simulink model "Motor_Model"  (R2025b)
settings: Solver=VariableStepAuto  StartTime=0.0  StopTime=2  RelTol=1e-3
undefined symbols (not defined in the file): c, J1, J2, k, ke, km, L, Mc, Ms, R

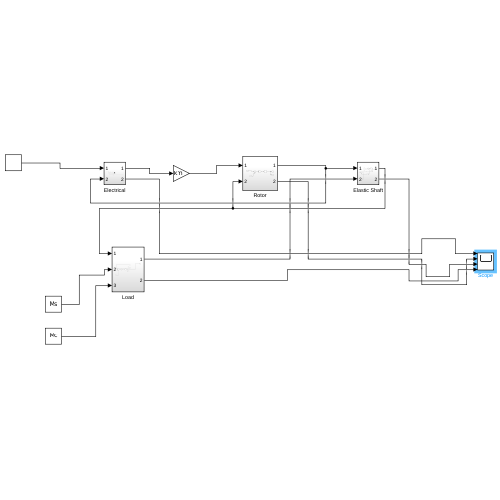
[thumbnail: Simulink's stored preview of the top-level diagram]
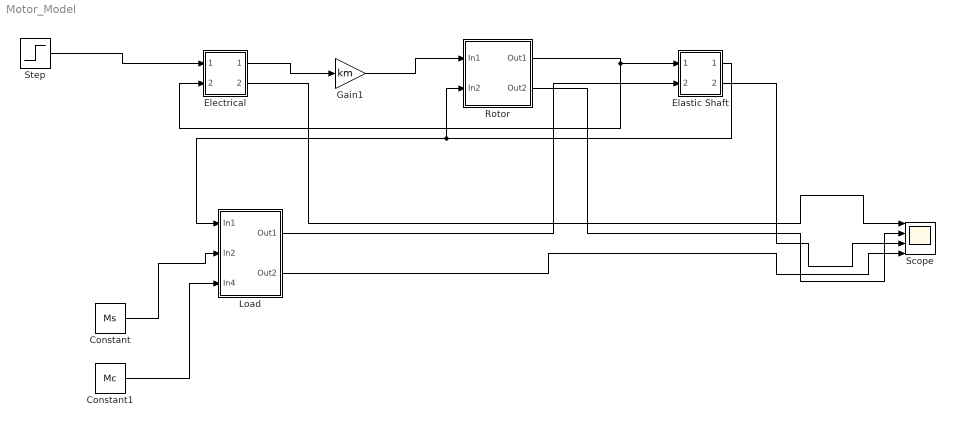
== system Motor_Model ==
  Constant : Constant  Value=Ms
  Constant1 : Constant  Value=Mc
  Elastic Shaft : Subsystem
  Electrical : Subsystem
  Gain1 : Gain  Gain=km
  Load : Subsystem
  Rotor : Subsystem
  Scope : Scope  NumInputPorts=4
      settings: ActiveDisplayYMinimum=-1.1593735821499702  ActiveDisplayYMaximum=10.434362239349735
  Step : Step  Time=0  After=24  SampleTime=0
  wires:
  Step/1 -> Electrical/1(In1)
  Electrical/1(Out1) -> Gain1/1
  Rotor/1(Out1) -> Electrical/2(In2), Elastic Shaft/1(In1)
  Gain1/1 -> Rotor/1(In1)
  Elastic Shaft/1(Out1) -> Load/1(In1), Rotor/2(In2)
  Load/1(Out1) -> Elastic Shaft/2(In2)
  Constant/1 -> Load/2(In2)
  Constant1/1 -> Load/3(In4)
  Electrical/2(Out2) -> Scope/1
  Rotor/2(Out2) -> Scope/2
  Elastic Shaft/2(Out3) -> Scope/3
  Load/2(Out2) -> Scope/4

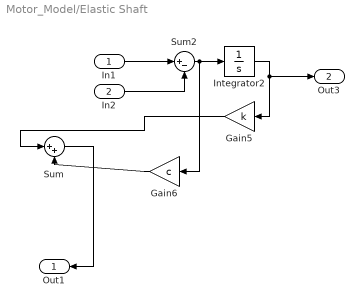
== system Motor_Model/Elastic Shaft ==
  In1 : Inport
  In2 : Inport  Port=2
  Gain5 : Gain  Gain=k
  Gain6 : Gain  Gain=c
  Integrator2 : Integrator
  Sum : Sum  Inputs=|++
  Sum2 : Sum  Inputs=|+-
  Out1 : Outport
  Out3 : Outport  Port=2
  wires:
  Sum2/1 -> Gain6/1, Integrator2/1
  In1/1 -> Sum2/1
  Integrator2/1 -> Out3/1, Gain5/1
  In2/1 -> Sum2/2
  Gain6/1 -> Sum/2
  Sum/1 -> Out1/1
  Gain5/1 -> Sum/1

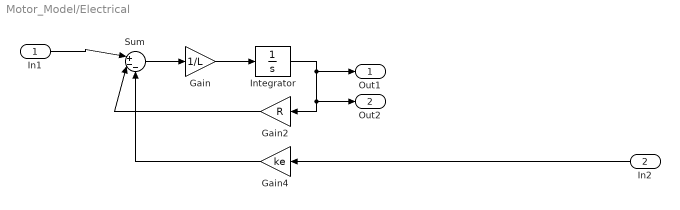
== system Motor_Model/Electrical ==
  In1 : Inport
  In2 : Inport  Port=2
  Gain : Gain  Gain=1/L
  Gain2 : Gain  Gain=R
  Gain4 : Gain  Gain=ke
  Integrator : Integrator
  Sum : Sum  Inputs=|+--
  Out1 : Outport
  Out2 : Outport  Port=2
  wires:
  Gain2/1 -> Sum/2
  Gain4/1 -> Sum/3
  Sum/1 -> Gain/1
  Gain/1 -> Integrator/1
  In2/1 -> Gain4/1
  In1/1 -> Sum/1
  Integrator/1 -> Gain2/1, Out2/1, Out1/1

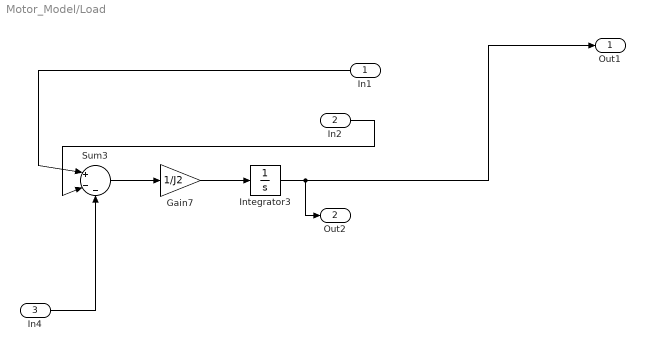
== system Motor_Model/Load ==
  In1 : Inport
  In2 : Inport  Port=2
  In4 : Inport  Port=3
  Gain7 : Gain  Gain=1/J2
  Integrator3 : Integrator
  Sum3 : Sum  Inputs=|+--
  Out1 : Outport
  Out2 : Outport  Port=2
  wires:
  Sum3/1 -> Gain7/1
  Gain7/1 -> Integrator3/1
  In4/1 -> Sum3/3
  Integrator3/1 -> Out2/1, Out1/1
  In1/1 -> Sum3/1
  In2/1 -> Sum3/2

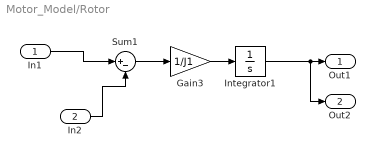
== system Motor_Model/Rotor ==
  In1 : Inport
  In2 : Inport  Port=2
  Gain3 : Gain  Gain=1/J1
  Integrator1 : Integrator
  Sum1 : Sum  Inputs=|+-
  Out1 : Outport
  Out2 : Outport  Port=2
  wires:
  Sum1/1 -> Gain3/1
  Gain3/1 -> Integrator1/1
  Integrator1/1 -> Out2/1, Out1/1
  In2/1 -> Sum1/2
  In1/1 -> Sum1/1
